simulink model "s1b"  (Simulink 2.00)
settings: Solver=ode45  StartTime=0.0  StopTime=tstop  MaxStep=1e-3  RelTol=1e-5  AbsTol=1e-5
values from neighbouring files (symbols this model uses):
  Psi1o = 0    [M1.M]    (also in M4.M)
  Psip2o = 0    [M1.M]    (also in M4.M)
  r1 = 0.25    [M1.M]    (also in M4.M)
  rp2 = 0.134    [M1.M]    (also in M4.M)
  wb = 2*pi*Frated    (= 376.991118431)    [M1.M]    (also in M4.M)
  xl1 = 0.056    [M1.M]    (also in M4.M)
  xM = 1/(1/xm + 1/xl1 + 1/xpl2)    (= 0.0279988939489)    [M1.M]    (also in M4.M)
  xm = 708.8    [M1.M]    (also in M4.M)
  xpl2 = 0.056    [M1.M]    (also in M4.M)
settings Model: SaveTime=off  SaveOutput=off  ConsistencyChecking=off

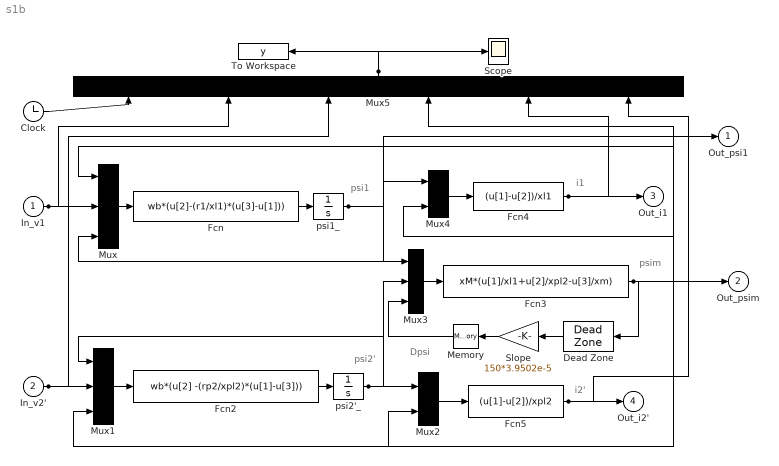
== system s1b ==
  note: i1
  note: psi1
  note: Dpsi
  note: psi2'
  note: i2'
  note: psim
  In_v1 : Inport  Port=1  PortWidth=-1  SampleTime=-1
  In_v2' : Inport  Port=2  PortWidth=-1  SampleTime=-1
  Clock : Clock
      settings: DeleteFcn=simclock BlockIsBeingDestroyed  PostSaveFcn=simclock Save
  Dead Zone : DeadZone  Orientation=left  LowerValue=-154  UpperValue=154
  Fcn : Fcn  Expr=wb*(u[2]-(r1/xl1)*(u[3]-u[1]))
  Fcn2 : Fcn  Expr=wb*(u[2] -(rp2/xpl2)*(u[1]-u[3]))
  Fcn3 : Fcn  Expr=xM*(u[1]/xl1+u[2]/xpl2-u[3]/xm)
  Fcn4 : Fcn  Expr=(u[1]-u[2])/xl1
  Fcn5 : Fcn  Expr=(u[1]-u[2])/xpl2
  Memory : Memory  Orientation=left  X0=0  InheritSampleTime=off
  Mux : Mux  Inputs=3
  Mux1 : Mux  Inputs=3
  Mux2 : Mux  Inputs=2
  Mux3 : Mux  Inputs=3
  Mux4 : Mux  Inputs=2
  Mux5 : Mux  Orientation=up  Inputs=6
  Scope : Scope
      settings: TickLabels=on  TimeRange=0.2  YMin=-300  YMax=300  SaveToWorkspace=off  SaveName=ScopeData  LimitMaxRows=off
  Slope : Gain  Orientation=left  Gain=150*3.9502e-5
  To Workspace : ToWorkspace  VariableName=y  SampleTime=0
      settings: Buffer=80000
  psi1_ : Integrator  ExternalReset=none  InitialConditionSource=internal  InitialCondition=Psi1o  LimitOutput=off  UpperSaturationLimit=inf  LowerSaturationLimit=-inf  ShowSaturationPort=off  ShowStatePort=off  AbsoluteTolerance=auto
  psi2'_ : Integrator  ExternalReset=none  InitialConditionSource=internal  InitialCondition=Psip2o  LimitOutput=off  UpperSaturationLimit=inf  LowerSaturationLimit=-inf  ShowSaturationPort=off  ShowStatePort=off  AbsoluteTolerance=auto
  Out_psi1 : Outport  Port=1  InitialOutput=0
  Out_psim : Outport  Port=2  InitialOutput=0
  Out_i1 : Outport  Port=3  InitialOutput=0
  Out_i2' : Outport  Port=4  InitialOutput=0
  wires:
  Mux/1 -> Fcn/1
  Fcn/1 -> psi1_/1
  Fcn2/1 -> psi2'_/1
  Mux3/1 -> Fcn3/1
  Mux4/1 -> Fcn4/1
  psi1_/1 -> Mux3/1, Mux4/1, Out_psi1/1, Mux/3
  Fcn3/1 -> Mux4/2, Mux1/3, Mux/1, Out_psim/1, Mux2/2, Mux5/4, Dead Zone/1
  Mux1/1 -> Fcn2/1
  psi2'_/1 -> Mux1/1, Mux3/2, Mux2/1
  Mux2/1 -> Fcn5/1
  In_v2'/1 -> Mux1/2, Mux5/3
  In_v1/1 -> Mux/2, Mux5/2
  Clock/1 -> Mux5/1
  Fcn4/1 -> Out_i1/1, Mux5/5
  Fcn5/1 -> Out_i2'/1, Mux5/6
  Mux5/1 -> Scope/1, To Workspace/1
  Dead Zone/1 -> Slope/1
  Slope/1 -> Memory/1
  Memory/1 -> Mux3/3
